simulink model "BatterySOC_CoulombCounting"  (R2025a)
settings: Solver=VariableStepAuto  StartTime=0.0  StopTime=3600*3  RelTol=1e-3
undefined symbols (not defined in the file): Ion, Lithium
libraries: spsBatteryLib x1, spsCurrentMeasurementLib x1, spsDCMachineLib x1, sps_lib x1
settings Model: Creator=Dell  LastModifiedBy=Dell

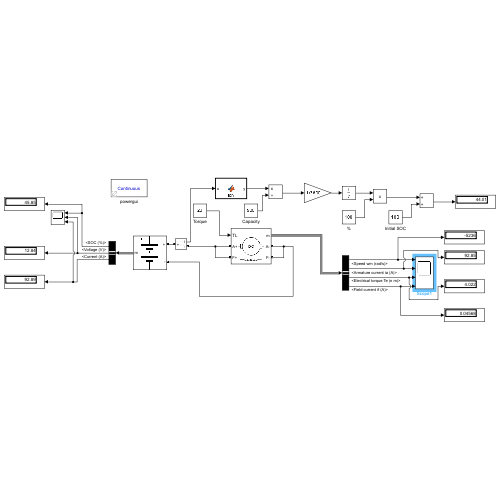
[thumbnail: Simulink's stored preview of the top-level diagram]
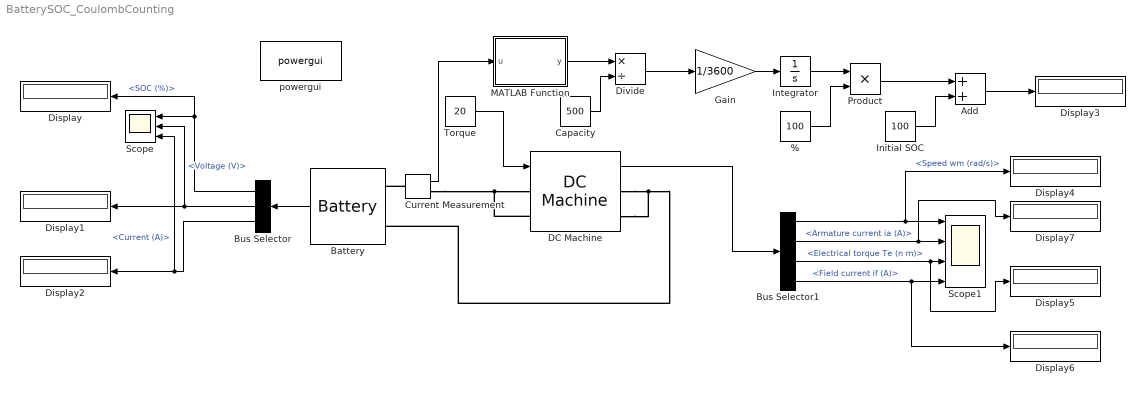
== system BatterySOC_CoulombCounting ==
  % : Constant  Value=100
  Add : Sum
  Battery : spsBatteryLib/Battery  BatType=Lithium-Ion  NomV=12  NomQ=500  SOC=100  Batt_Tr=30  PresetModel=on  MaxQ=500  MinV=9  FullV=13.9678  Dis_rate=217.3913  R=0.00024  Normal_OP=452.1739  expZone="[12.9646      24.5652]"
  Bus Selector : BusSelector  OutputSignals=SOC (%),Voltage (V),Current (A)
  Bus Selector1 : BusSelector  OutputSignals=Speed wm (rad/s),Armature current ia (A),Electrical torque Te (n m),Field current if (A)
  Capacity : Constant  Value=500
  Current Measurement : spsCurrentMeasurementLib/Current Measurement  PhasorSimulation=off  OutputType=Complex  PSBequivalent=0
  DC Machine : spsDCMachineLib/DC Machine  PresetModel=01: 5HP 240V 1750RPM Field:300V  MechanicalLoad=Torque TL  FieldType=Wound  ShowDetailedParameters=on  MeasurementBus=off  RLa=[2.581 0.028]  RLf=[281.2 156]  Laf=0.9483  MachineConstant=Torque constant (N.m/A)  Ke=1.8  Kt=1.8  J=0.02215  Bm=0.002953  Tf=0.5161  w0=1  Ifinit=0  TsPowergui=0  TsBlock=-1
  Display{,1..7} (8 alike) : Display
  Divide : Product  Inputs=*/
  Gain : Gain  Gain=1/3600
  Initial SOC : Constant  Value=100
  Integrator : Integrator
  MATLAB Function : MATLAB Function  TreatAsAtomicUnit=on
  Product : Product
  Scope : Scope  NumInputPorts=3
      settings: ActiveDisplayYMinimum=-12.499999999999996  ActiveDisplayYMaximum=112.5
  Scope1 : Scope  NumInputPorts=4
      settings: ActiveDisplayYMinimum=-5902.7302913957765  ActiveDisplayYMaximum=763.56275400750565
  Torque : Constant  Value=20
  powergui : sps_lib/powergui  Priority=1  SimulationMode=Continuous  SampleTime=50e-6  frequency=60  Iterations=50  frequencyindice=0  Pbase=100e6  ErrMax=1e-4  UnitsV=kV  UnitsW=MW  buscounter=0  FunctionMessages=off  echomessages=off  EnableUseOfTLC=off  CurrentSourceSwitches=off  DisableSnubberDevices=off  DisableRonSwitches=off  DisableVfSwitches=off  DisplayEquations=off  AutomaticDiscreteSolvers=off  SolverType=Tustin/Backward Euler (TBE)  Interpol=off  ExternalGateDelay=off  methode=off  Ts=100  x0status=blocks  SPID=on  SwTol=0  HookPort=off  NonlinearTolerance=1e-4  nMaxIteration=100  ContinueOnMaxIteration=off  RestoreLinks=warning  ResistiveCurrentMeasurement=off  Frange=[0:2:500]  Ylog=off  Xlog=on  ShowGrid=off  save=off  variable=ZData  structure=0  ZoomFFT=off  StartTime=0.0  cycles=1  DisplayStyle=1  fundamental=60  FreqAxis=off  MaxFrequency=1000  frequencyindicesteady=1  RmsSteady=1  display=off
  wires:
  Battery/1 -> Bus Selector/1
  Bus Selector/1 -> Display/1, Scope/1  "<SOC (%)>"
  Bus Selector/2 -> Scope/2, Display1/1  "<Voltage (V)>"
  Bus Selector/3 -> Display2/1, Scope/3  "<Current (A)>"
  Torque/1 -> DC Machine/1
  Current Measurement/1 -> MATLAB Function/1(u)
  MATLAB Function/1(y) -> Divide/1
  Capacity/1 -> Divide/2
  Divide/1 -> Gain/1
  Gain/1 -> Integrator/1
  Integrator/1 -> Product/1
  %/1 -> Product/2
  Product/1 -> Add/1
  Initial SOC/1 -> Add/2
  Add/1 -> Display3/1
  DC Machine/1 -> Bus Selector1/1
  Bus Selector1/1 -> Scope1/1, Display4/1  "<Speed wm (rad/s)>"
  Bus Selector1/2 -> Scope1/2, Display7/1  "<Armature current ia (A)>"
  Bus Selector1/3 -> Display5/1, Scope1/3  "<Electrical torque Te (n m)>"
  Bus Selector1/4 -> Scope1/4, Display6/1  "<Field current if (A)>"
  connections:
  DC Machine/RConn1 -- DC Machine/RConn2 -- Battery/LConn2
  Current Measurement/LConn1 -- Battery/LConn1
  Current Measurement/RConn1 -- DC Machine/LConn2 -- DC Machine/LConn1

== matlab function BatterySOC_CoulombCounting/MATLAB Function ==
  data: u input; y output
function y = fcn(u)

y = -u;
